simulink model "X4_CentraInver"  (R2024b)
settings: Solver=VariableStepAuto  StartTime=0.0  StopTime=20  RelTol=1e-3
libraries: Mako_Dynamics x2
settings Model: Creator=pinto  LastModifiedBy=pinto

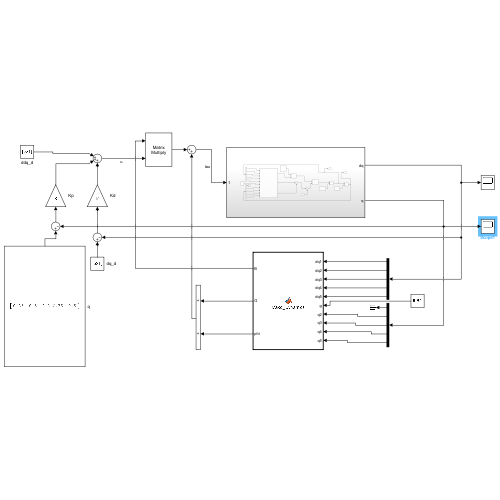
[thumbnail: Simulink's stored preview of the top-level diagram]
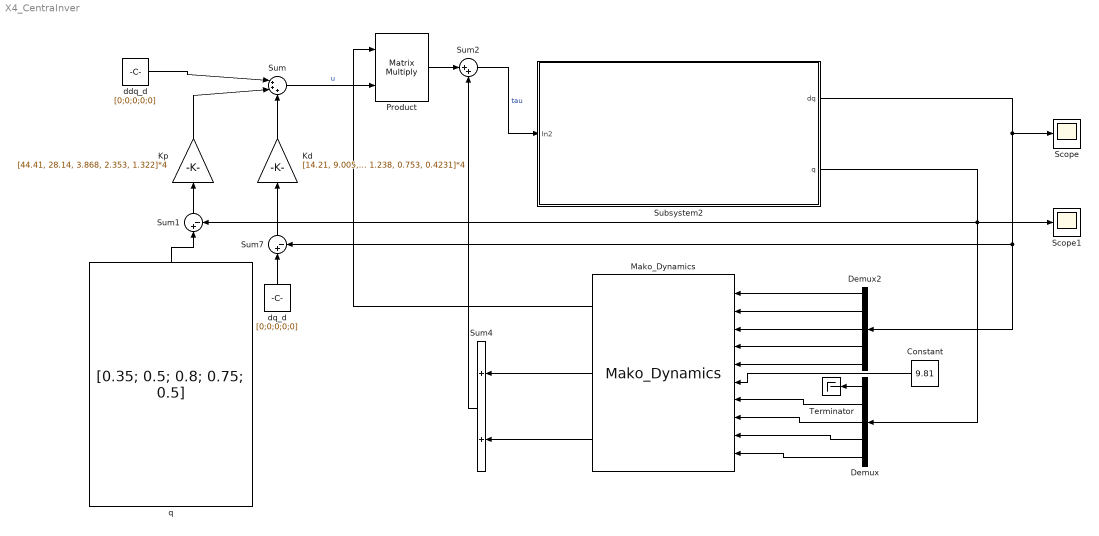
== system X4_CentraInver ==
  Constant : Constant  Value=9.81
  Demux : Demux  Outputs=5
  Demux2 : Demux  Outputs=5
  Kd : Gain  Gain=[14.21, 9.005, 1.238, 0.753, 0.4231]*4
  Kp : Gain  Gain=[44.41, 28.14, 3.868, 2.353, 1.322]*4
  Mako_Dynamics : Mako_Dynamics/Mako_Dynamics  SystemSampleTime=-1  VariantActivationTime=update diagram  AllowFlexibleInterface=on  Latency=0  AutoFrameSizeCalculation=off
  Product : Product  Multiplication=Matrix(*)
  Scope : Scope
  Scope1 : Scope
  Subsystem2 : Subsystem
  Sum : Sum  Inputs=|+++
  Sum1 : Sum  Inputs=|+-
  Sum2 : Sum  Inputs=|++
  Sum4 : Sum
  Sum7 : Sum  Inputs=|+-
  Terminator : Terminator
  ddq_d : Constant  Value=[0;0;0;0;0]
  dq_d : Constant  Value=[0;0;0;0;0]
  q : Constant  Value=[0.35; 0.5; 0.8; 0.75; 0.5]
  wires:
  Sum/1 -> Product/2  "u"
  Kd/1 -> Sum/3
  Subsystem2/2(q) -> Scope1/1, Sum1/2, Demux/1
  Product/1 -> Sum2/1
  Kp/1 -> Sum/2
  Sum4/1 -> Sum2/2
  dq_d/1 -> Sum7/1
  Subsystem2/1(dq) -> Demux2/1, Sum7/2, Scope/1
  Sum7/1 -> Kd/1
  Sum2/1 -> Subsystem2/1(In2)  "tau"
  Demux2/4 -> Mako_Dynamics/4
  Demux2/1 -> Mako_Dynamics/1
  Demux2/3 -> Mako_Dynamics/3
  Demux2/2 -> Mako_Dynamics/2
  Mako_Dynamics/1 -> Product/1
  Demux2/5 -> Mako_Dynamics/5
  Mako_Dynamics/2 -> Sum4/1
  Mako_Dynamics/3 -> Sum4/2
  Demux/1 -> Terminator/1
  Sum1/1 -> Kp/1
  q/1 -> Sum1/1
  ddq_d/1 -> Sum/1
  Demux/2 -> Mako_Dynamics/7
  Demux/3 -> Mako_Dynamics/8
  Demux/4 -> Mako_Dynamics/9
  Demux/5 -> Mako_Dynamics/10
  Constant/1 -> Mako_Dynamics/6

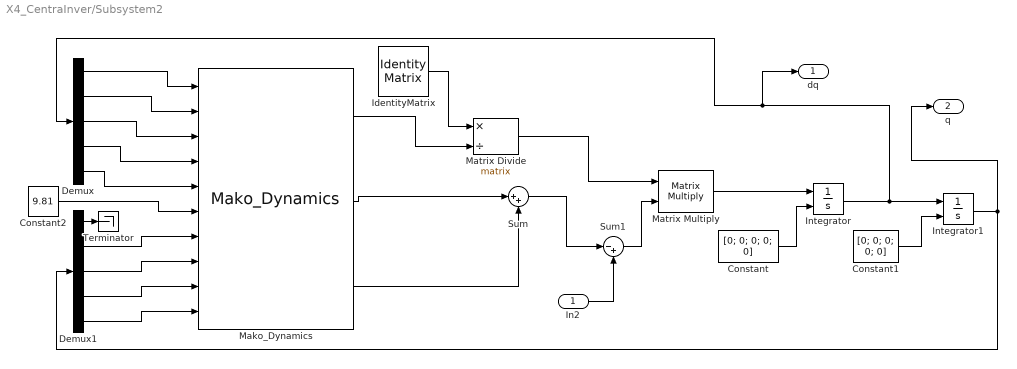
== system X4_CentraInver/Subsystem2 ==
  In2 : Inport
  Constant : Constant  Value=[0; 0; 0; 0; 0]
  Constant1 : Constant  Value=[0; 0; 0; 0; 0]
  Constant2 : Constant  Value=9.81
  Demux : Demux  Outputs=5
  Demux1 : Demux  Outputs=5
  IdentityMatrix : IdentityMatrix
  Integrator : Integrator  InitialConditionSource=external  InitialCondition=[0.01, 0.01, 0.01]
  Integrator1 : Integrator  InitialConditionSource=external  InitialCondition=[0.01, 0.01, 0.01]
  Mako_Dynamics : Mako_Dynamics/Mako_Dynamics  SystemSampleTime=-1  VariantActivationTime=update diagram  AllowFlexibleInterface=on  Latency=0  AutoFrameSizeCalculation=off
  Matrix Divide : Product  Inputs=*/  Multiplication=Matrix(*)
  Matrix Multiply : Product  Multiplication=Matrix(*)
  Sum : Sum  Inputs=|++
  Sum1 : Sum  Inputs=|-+
  Terminator : Terminator
  dq : Outport
  q : Outport  Port=2
  wires:
  Sum/1 -> Sum1/1
  Demux/3 -> Mako_Dynamics/3
  IdentityMatrix/1 -> Matrix Divide/1
  Integrator/1 -> Integrator1/1, Demux/1, dq/1
  Matrix Multiply/1 -> Integrator/1
  Demux/4 -> Mako_Dynamics/4
  Demux/2 -> Mako_Dynamics/2
  Constant1/1 -> Integrator1/2
  Integrator1/1 -> q/1, Demux1/1
  Mako_Dynamics/1 -> Matrix Divide/2
  Matrix Divide/1 -> Matrix Multiply/1
  Constant/1 -> Integrator/2
  Sum1/1 -> Matrix Multiply/2
  Demux/1 -> Mako_Dynamics/1
  In2/1 -> Sum1/2
  Demux/5 -> Mako_Dynamics/5
  Mako_Dynamics/2 -> Sum/1
  Mako_Dynamics/3 -> Sum/2
  Demux1/1 -> Terminator/1
  Constant2/1 -> Mako_Dynamics/6
  Demux1/2 -> Mako_Dynamics/7
  Demux1/3 -> Mako_Dynamics/8
  Demux1/4 -> Mako_Dynamics/9
  Demux1/5 -> Mako_Dynamics/10
